simulink model "EE401_Lab_Simulation_DQ Frame"  (R2019a)
settings: Solver=VariableStepAuto  StartTime=0.0  StopTime=2  MaxStep=0.0001  RelTol=1e-3
model workspace (MAT data in the model file):
  J = 0.02
  Lm = 0.2037
  Lr = 0.2097
  Ls = 0.2097
  P = 4
  Rr = 1.083
  Rs = 1.115
  TL = 20
  We = 376.99
libraries: powerlib x1
settings Model: OrderedModelArguments=off  Creator=omkar  LastModifiedBy=omkar

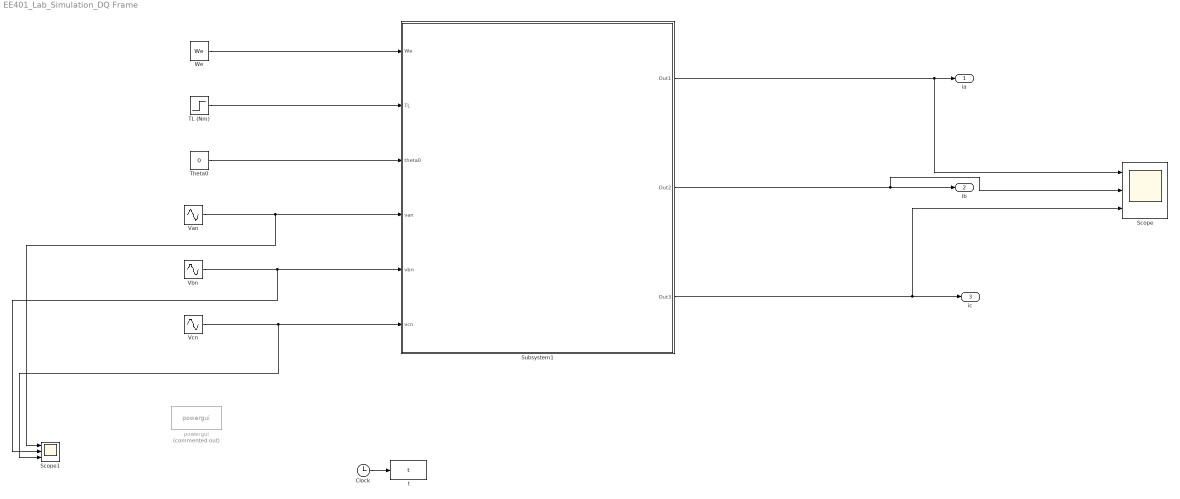
== system EE401_Lab_Simulation_DQ Frame ==
  "Clock " : Clock
  Scope : Scope  NumInputPorts=3
  Scope1 : Scope  NumInputPorts=3
  Subsystem1 : Subsystem
  TL (Nm) : Step  Time=0.2  After=TL  SampleTime=0
  Theta0 : Constant  Value=0
  Van : Sin  Amplitude=240  Frequency=2*pi*60  SampleTime=0
  Vbn : Sin  Amplitude=240  Frequency=2*pi*60  Phase=-2*pi/3  SampleTime=0
  Vcn : Sin  Amplitude=240  Frequency=2*pi*60  Phase=-4*pi/3  SampleTime=0
  We : Constant  Value=We
  powergui : powerlib/powergui  Priority=1  Commented=on  SimulationMode=Continuous  SampleTime=50e-6  frequency=60  Iterations=50  frequencyindice=60  Pbase=100e6  ErrMax=1e-4  UnitsV=kV  UnitsW=MW  buscounter=0  FunctionMessages=off  echomessages=off  EnableUseOfTLC=off  CurrentSourceSwitches=off  DisableSnubberDevices=off  DisableRonSwitches=off  DisableVfSwitches=off  DisplayEquations=off  AutomaticDiscreteSolvers=off  SolverType=Tustin/Backward Euler (TBE)  Interpol=off  ExternalGateDelay=off  methode=off  Ts=100  x0status=blocks  SPID=on  SwTol=0  HookPort=off  NonlinearTolerance=0  nMaxIteration=15  ContinueOnMaxIteration=off  RestoreLinks=warning  ResistiveCurrentMeasurement=off  Frange=[0:2:500]  Ylog=off  Xlog=on  ShowGrid=off  save=off  variable=ZData  structure=0  ZoomFFT=off  StartTime=0.0  cycles=1  DisplayStyle=1  fundamental=60  FreqAxis=off  MaxFrequency=1000  frequencyindicesteady=1  RmsSteady=1  display=off
      settings: SourceProductName=Simscape Electrical
  t : ToWorkspace  VariableName=t  SaveFormat=Timeseries  SampleTime=-1
  ia : Outport  VectorParamsAs1DForOutWhenUnconnected=on
  ib : Outport  Port=2  VectorParamsAs1DForOutWhenUnconnected=on
  ic : Outport  Port=3  VectorParamsAs1DForOutWhenUnconnected=on
  wires:
  We/1 -> Subsystem1/1(We)
  Theta0/1 -> Subsystem1/3(theta0)
  Subsystem1/1(Out1) -> Scope/1, ia/1
  Subsystem1/2(Out2) -> Scope/2, ib/1
  Subsystem1/3(Out3) -> Scope/3, ic/1
  Van/1 -> Scope1/1, Subsystem1/4(van)
  Vbn/1 -> Scope1/2, Subsystem1/5(vbn)
  Vcn/1 -> Scope1/3, Subsystem1/6(vcn)
  TL (Nm)/1 -> Subsystem1/2(TL)
  "Clock "/1 -> t/1

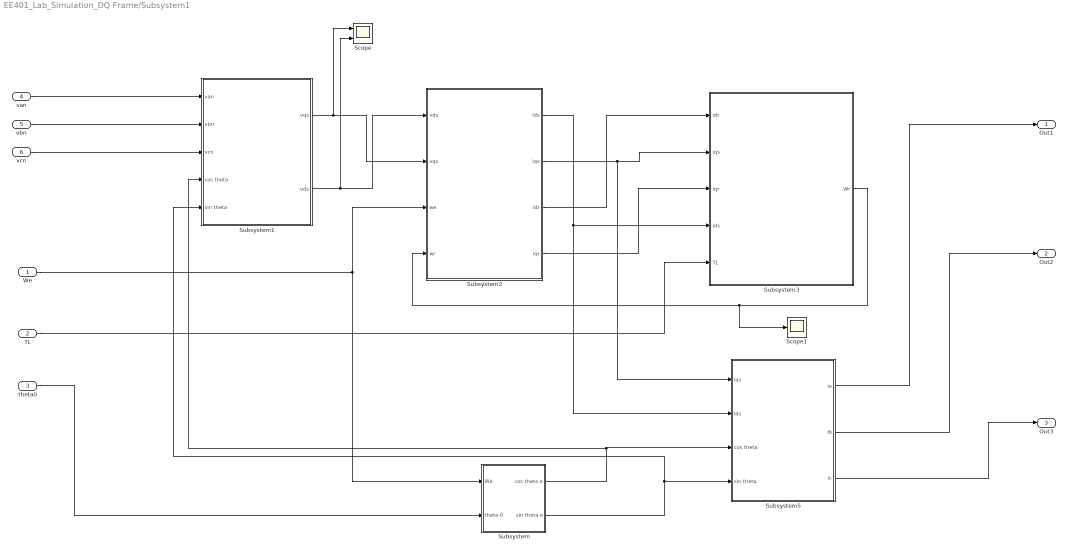
== system EE401_Lab_Simulation_DQ Frame/Subsystem1 ==
  We : Inport
  TL : Inport  Port=2
  theta0 : Inport  Port=3
  van : Inport  Port=4
  vbn : Inport  Port=5
  vcn : Inport  Port=6
  Scope : Scope  NumInputPorts=2
  Scope1 : Scope
  Subsystem : Subsystem
  Subsystem1 : Subsystem
  Subsystem2 : Subsystem
  Subsystem3 : Subsystem
  Subsystem5 : Subsystem
  Out1 : Outport
  Out2 : Outport  Port=2
  Out3 : Outport  Port=3
  wires:
  Subsystem5/3(ic) -> Out3/1
  We/1 -> Subsystem2/3(we), Subsystem/1(We)
  Subsystem2/4(iqr) -> Subsystem3/3(iqr)
  Subsystem2/3(idr) -> Subsystem3/1(idr)
  Subsystem2/1(ids) -> Subsystem5/2(ids), Subsystem3/4(ids)
  Subsystem2/2(iqs) -> Subsystem5/1(iqs), Subsystem3/2(iqs)
  Subsystem3/1(Wr) -> Scope1/1, Subsystem2/4(wr)
  Subsystem5/1(ia) -> Out1/1
  Subsystem5/2(ib) -> Out2/1
  theta0/1 -> Subsystem/2(theta 0)
  TL/1 -> Subsystem3/5(TL)
  Subsystem1/2(vds) -> Scope/2, Subsystem2/1(vds)
  Subsystem1/1(vqs) -> Scope/1, Subsystem2/2(vqs)
  van/1 -> Subsystem1/1(van)
  vbn/1 -> Subsystem1/2(vbn)
  vcn/1 -> Subsystem1/3(vcn)
  Subsystem/1(cos theta e) -> Subsystem1/4(cos theta), Subsystem5/3(cos theta)
  Subsystem/2(sin theta e) -> Subsystem5/4(sin theta), Subsystem1/5(sin theta)

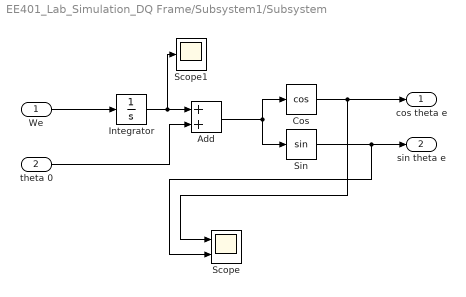
== system EE401_Lab_Simulation_DQ Frame/Subsystem1/Subsystem ==
  We : Inport
  theta 0 : Inport  Port=2
  Add : Sum
  Cos : Trigonometry  Operator=cos
  Integrator : Integrator
  Scope : Scope  NumInputPorts=2
  Scope1 : Scope
  Sin : Trigonometry
  cos theta e : Outport
  sin theta e : Outport  Port=2
  wires:
  Integrator/1 -> Scope1/1, Add/1
  Add/1 -> Cos/1, Sin/1
  theta 0/1 -> Add/2
  Sin/1 -> Scope/2, sin theta e/1
  We/1 -> Integrator/1
  Cos/1 -> Scope/1, cos theta e/1

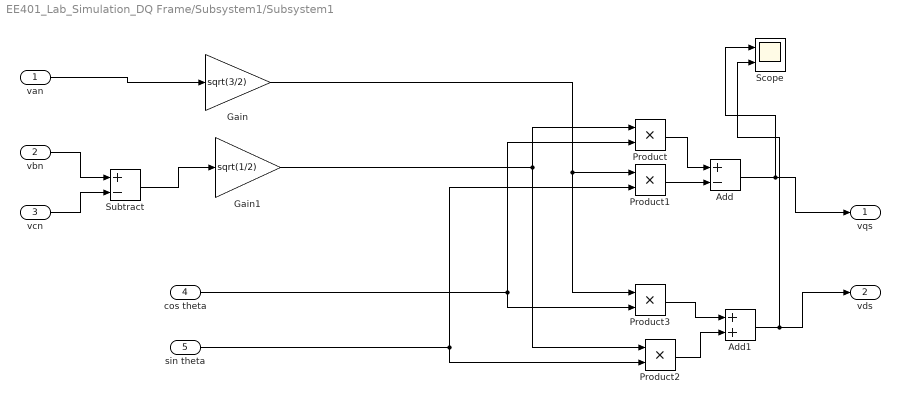
== system EE401_Lab_Simulation_DQ Frame/Subsystem1/Subsystem1 ==
  van : Inport
  vbn : Inport  Port=2
  vcn : Inport  Port=3
  cos theta : Inport  Port=4
  sin theta : Inport  Port=5
  Add : Sum  Inputs=+-
  Add1 : Sum
  Gain : Gain  Gain=sqrt(3/2)
  Gain1 : Gain  Gain=sqrt(1/2)
  Product{,1..3} (4 alike) : Product
  Scope : Scope  NumInputPorts=2
  Subtract : Sum  Inputs=+-
  vqs : Outport
  vds : Outport  Port=2
  wires:
  van/1 -> Gain/1
  sin theta/1 -> Product2/2, Product1/2
  Product1/1 -> Add/2
  cos theta/1 -> Product/2, Product3/2
  Gain/1 -> Product1/1, Product3/1
  Product2/1 -> Add1/2
  Product3/1 -> Add1/1
  Product/1 -> Add/1
  Gain1/1 -> Product/1, Product2/1
  vbn/1 -> Subtract/1
  vcn/1 -> Subtract/2
  Add/1 -> Scope/1, vqs/1
  Add1/1 -> Scope/2, vds/1
  Subtract/1 -> Gain1/1

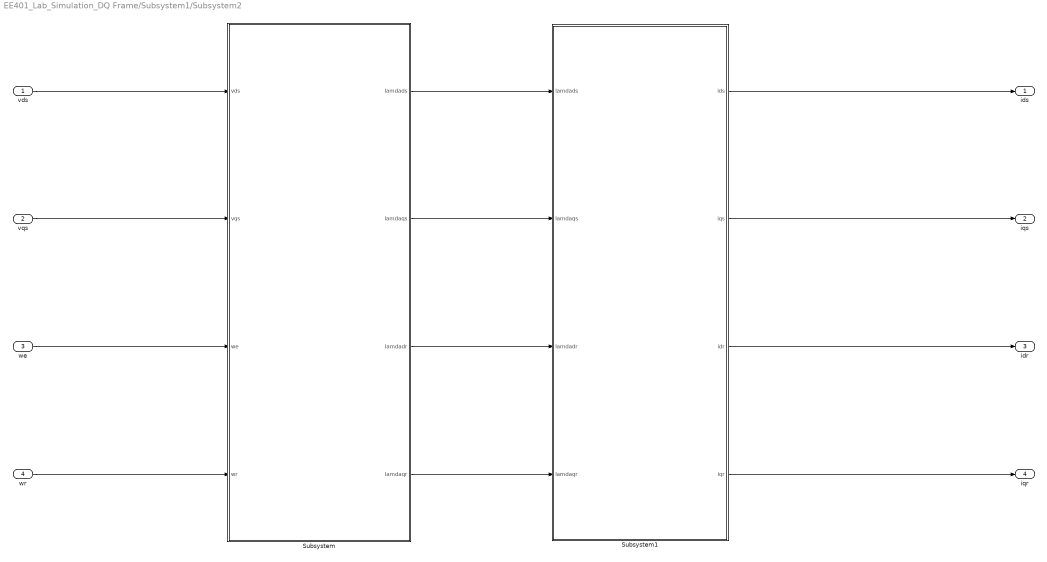
== system EE401_Lab_Simulation_DQ Frame/Subsystem1/Subsystem2 ==
  vds : Inport
  vqs : Inport  Port=2
  we : Inport  Port=3
  wr : Inport  Port=4
  Subsystem : Subsystem
  Subsystem1 : Subsystem
  ids : Outport
  iqs : Outport  Port=2
  idr : Outport  Port=3
  iqr : Outport  Port=4
  wires:
  wr/1 -> Subsystem/4(wr)
  Subsystem1/3(idr) -> idr/1
  Subsystem/4(lamdaqr) -> Subsystem1/4(lamdaqr)
  Subsystem/3(lamdadr) -> Subsystem1/3(lamdadr)
  Subsystem/1(lamdads) -> Subsystem1/1(lamdads)
  we/1 -> Subsystem/3(we)
  Subsystem/2(lamdaqs) -> Subsystem1/2(lamdaqs)
  Subsystem1/4(iqr) -> iqr/1
  Subsystem1/1(ids) -> ids/1
  Subsystem1/2(iqs) -> iqs/1
  vds/1 -> Subsystem/1(vds)
  vqs/1 -> Subsystem/2(vqs)

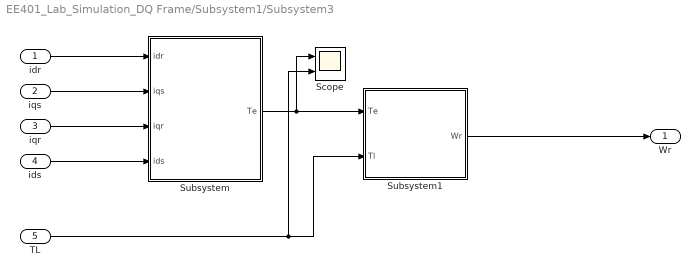
== system EE401_Lab_Simulation_DQ Frame/Subsystem1/Subsystem3 ==
  idr : Inport
  iqs : Inport  Port=2
  iqr : Inport  Port=3
  ids : Inport  Port=4
  TL : Inport  Port=5
  Scope : Scope  NumInputPorts=2
  Subsystem : Subsystem
  Subsystem1 : Subsystem
  Wr : Outport
  wires:
  ids/1 -> Subsystem/4(ids)
  iqr/1 -> Subsystem/3(iqr)
  Subsystem/1(Te) -> Scope/1, Subsystem1/1(Te)
  idr/1 -> Subsystem/1(idr)
  Subsystem1/1(Wr) -> Wr/1
  TL/1 -> Scope/2, Subsystem1/2(Tl)
  iqs/1 -> Subsystem/2(iqs)

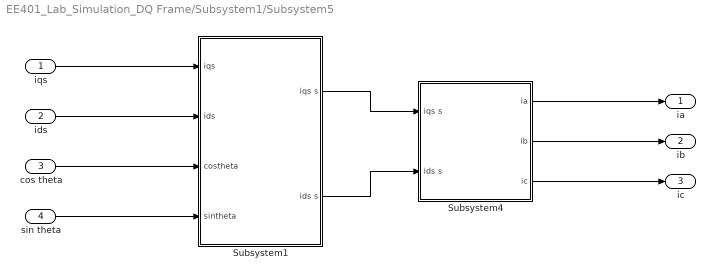
== system EE401_Lab_Simulation_DQ Frame/Subsystem1/Subsystem5 ==
  iqs : Inport
  ids : Inport  Port=2
  cos theta : Inport  Port=3
  sin theta : Inport  Port=4
  Subsystem1 : Subsystem
  Subsystem4 : Subsystem
  ia : Outport
  ib : Outport  Port=2
  ic : Outport  Port=3
  wires:
  sin theta/1 -> Subsystem1/4(sintheta)
  Subsystem1/1(iqs s) -> Subsystem4/1(iqs s)
  Subsystem4/1(ia) -> ia/1
  Subsystem4/3(ic) -> ic/1
  ids/1 -> Subsystem1/2(ids)
  cos theta/1 -> Subsystem1/3(costheta)
  Subsystem4/2(ib) -> ib/1
  Subsystem1/2(ids s) -> Subsystem4/2(ids s)
  iqs/1 -> Subsystem1/1(iqs)

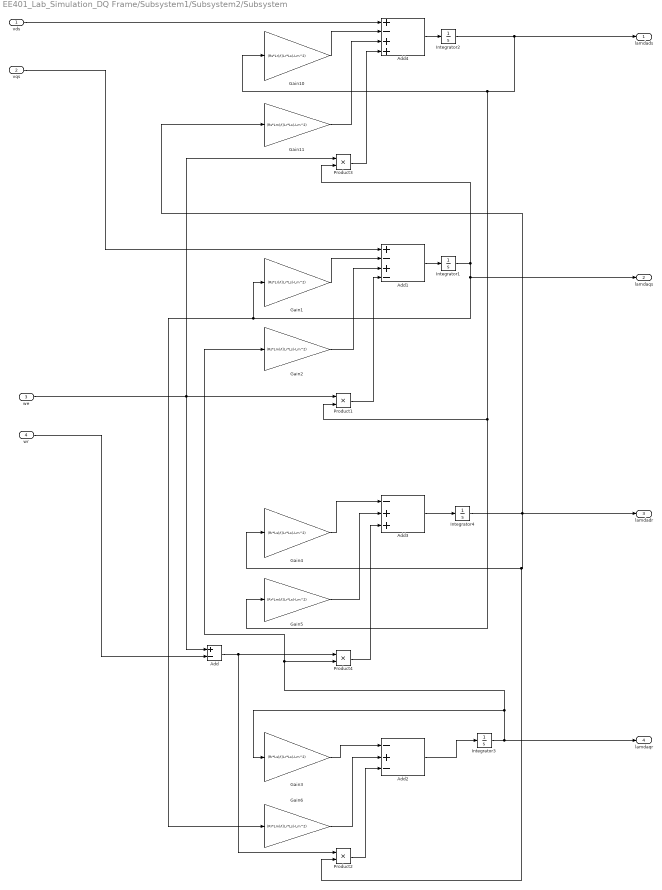
== system EE401_Lab_Simulation_DQ Frame/Subsystem1/Subsystem2/Subsystem ==
  vds : Inport
  vqs : Inport  Port=2
  we : Inport  Port=3
  wr : Inport  Port=4
  Add : Sum  Inputs=+-
  Add1 : Sum  Inputs=+-+-
  Add2 : Sum  Inputs=-+-
  Add3 : Sum  Inputs=-++
  Add4 : Sum  Inputs=+-++
  Gain1 : Gain  Gain=(Rs*Lr)/((Lr*Ls)-Lm^2)
  Gain10 : Gain  Gain=(Rs*Lr)/((Lr*Ls)-Lm^2)
  Gain11 : Gain  Gain=(Rs*Lm)/((Lr*Ls)-Lm^2)
  Gain2 : Gain  Gain=(Rs*Lm)/((Lr*Ls)-Lm^2)
  Gain3 : Gain  Gain=(Rr*Ls)/((Lr*Ls)-Lm^2)
  Gain4 : Gain  Gain=(Rr*Ls)/((Lr*Ls)-Lm^2)
  Gain5 : Gain  Gain=(Rr*Lm)/((Lr*Ls)-Lm^2)
  Gain6 : Gain  Gain=(Rr*Lm)/((Lr*Ls)-Lm^2)
  Integrator{1..4} (4 alike) : Integrator
  Product{1..4} (4 alike) : Product
  lamdads : Outport
  lamdaqs : Outport  Port=2
  lamdadr : Outport  Port=3
  lamdaqr : Outport  Port=4
  wires:
  Gain4/1 -> Add3/1
  Gain3/1 -> Add2/1
  Gain2/1 -> Add1/3
  Product2/1 -> Add2/3
  vqs/1 -> Add1/1
  Integrator1/1 -> lamdaqs/1, Gain6/1, Gain1/1, Product3/2
  Integrator2/1 -> lamdads/1, Gain10/1, Gain5/1, Product1/2
  we/1 -> Product3/1, Add/1, Product1/1
  Gain5/1 -> Add3/2
  Gain11/1 -> Add4/3
  Integrator4/1 -> Gain11/1, lamdadr/1, Product2/2, Gain4/1
  Product4/1 -> Add3/3
  Add2/1 -> Integrator3/1
  Gain6/1 -> Add2/2
  Add4/1 -> Integrator2/1
  Integrator3/1 -> lamdaqr/1, Gain2/1, Product4/2, Gain3/1
  Add3/1 -> Integrator4/1
  wr/1 -> Add/2
  Gain1/1 -> Add1/2
  Add1/1 -> Integrator1/1
  Product1/1 -> Add1/4
  Product3/1 -> Add4/4
  Gain10/1 -> Add4/2
  Add/1 -> Product4/1, Product2/1
  vds/1 -> Add4/1

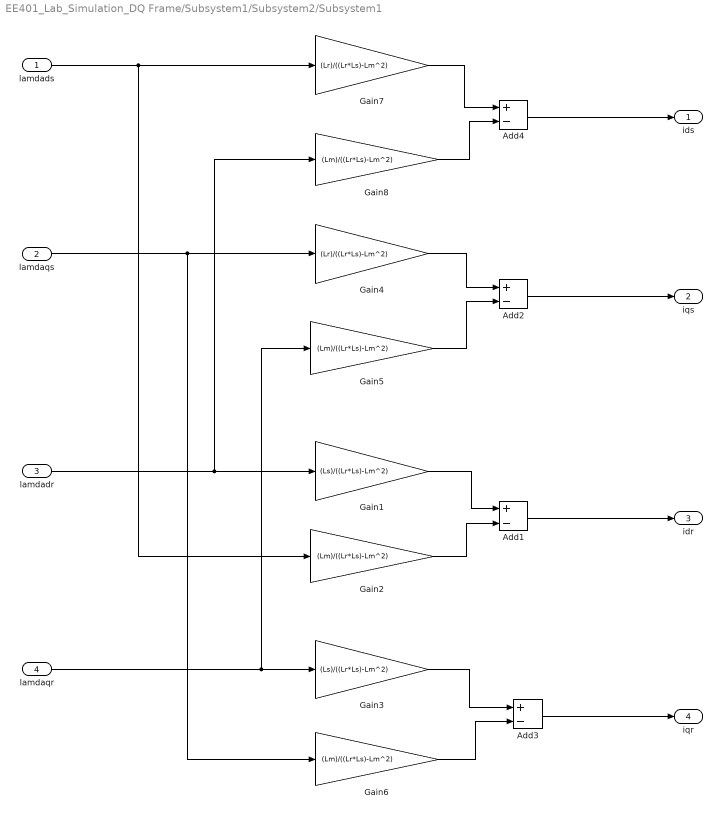
== system EE401_Lab_Simulation_DQ Frame/Subsystem1/Subsystem2/Subsystem1 ==
  lamdads : Inport
  lamdaqs : Inport  Port=2
  lamdadr : Inport  Port=3
  lamdaqr : Inport  Port=4
  Add{1..4} (4 alike) : Sum  Inputs=+-
  Gain1 : Gain  Gain=(Ls)/((Lr*Ls)-Lm^2)
  Gain{2,5..6,8} (4 alike) : Gain  Gain=(Lm)/((Lr*Ls)-Lm^2)
  Gain3 : Gain  Gain=(Ls)/((Lr*Ls)-Lm^2)
  Gain4 : Gain  Gain=(Lr)/((Lr*Ls)-Lm^2)
  Gain7 : Gain  Gain=(Lr)/((Lr*Ls)-Lm^2)
  ids : Outport
  iqs : Outport  Port=2
  idr : Outport  Port=3
  iqr : Outport  Port=4
  wires:
  Gain1/1 -> Add1/1
  Gain2/1 -> Add1/2
  Gain4/1 -> Add2/1
  Gain8/1 -> Add4/2
  Gain7/1 -> Add4/1
  Gain5/1 -> Add2/2
  lamdadr/1 -> Gain1/1, Gain8/1
  lamdaqs/1 -> Gain6/1, Gain4/1
  lamdaqr/1 -> Gain5/1, Gain3/1
  Add4/1 -> ids/1
  lamdads/1 -> Gain2/1, Gain7/1
  Gain6/1 -> Add3/2
  Gain3/1 -> Add3/1
  Add2/1 -> iqs/1
  Add1/1 -> idr/1
  Add3/1 -> iqr/1

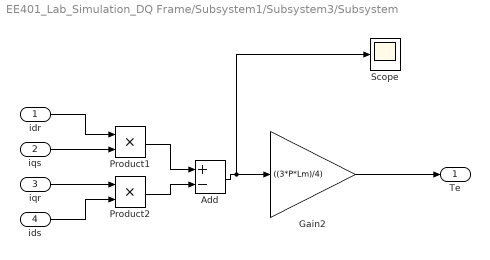
== system EE401_Lab_Simulation_DQ Frame/Subsystem1/Subsystem3/Subsystem ==
  idr : Inport
  iqs : Inport  Port=2
  iqr : Inport  Port=3
  ids : Inport  Port=4
  Add : Sum  Inputs=+-
  Gain2 : Gain  Gain=((3*P*Lm)/4)
  Product1 : Product
  Product2 : Product
  Scope : Scope
  Te : Outport
  wires:
  Product2/1 -> Add/2
  Product1/1 -> Add/1
  iqs/1 -> Product1/2
  iqr/1 -> Product2/1
  Gain2/1 -> Te/1
  Add/1 -> Scope/1, Gain2/1
  ids/1 -> Product2/2
  idr/1 -> Product1/1

== system EE401_Lab_Simulation_DQ Frame/Subsystem1/Subsystem3/Subsystem1 ==
  Te : Inport
  Tl : Inport  Port=2
  Add3 : Sum  Inputs=+-
  Gain6 : Gain  Gain=(P)/(2*J)
  Integrator1 : Integrator
  Scope1 : Scope  NumInputPorts=2
  Wr : Outport
  wires:
  Tl/1 -> Scope1/2, Add3/2
  Add3/1 -> Gain6/1
  Gain6/1 -> Integrator1/1
  Integrator1/1 -> Wr/1
  Te/1 -> Scope1/1, Add3/1

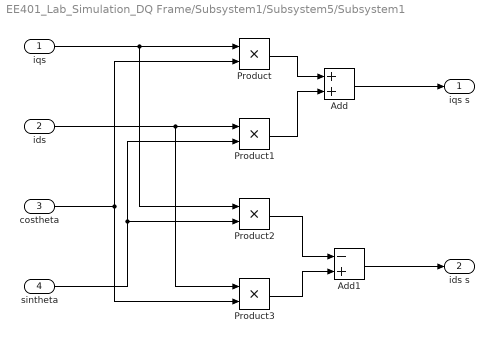
== system EE401_Lab_Simulation_DQ Frame/Subsystem1/Subsystem5/Subsystem1 ==
  iqs : Inport
  ids : Inport  Port=2
  costheta : Inport  Port=3
  sintheta : Inport  Port=4
  Add : Sum
  Add1 : Sum  Inputs=-+
  Product{,1..3} (4 alike) : Product
  iqs s : Outport
  ids s : Outport  Port=2
  wires:
  Product3/1 -> Add1/2
  costheta/1 -> Product/2, Product3/2
  sintheta/1 -> Product2/2, Product1/2
  Add/1 -> iqs s/1
  Product2/1 -> Add1/1
  iqs/1 -> Product2/1, Product/1
  Product1/1 -> Add/2
  Product/1 -> Add/1
  ids/1 -> Product3/1, Product1/1
  Add1/1 -> ids s/1

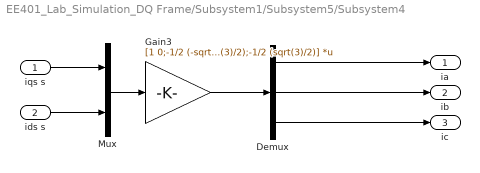
== system EE401_Lab_Simulation_DQ Frame/Subsystem1/Subsystem5/Subsystem4 ==
  iqs s : Inport
  ids s : Inport  Port=2
  Demux : Demux  Outputs=3
  Gain3 : Gain  Gain=[1 0;-1/2 (-sqrt(3)/2);-1/2 (sqrt(3)/2)]  Multiplication=Matrix(K*u)
  Mux : Mux  Inputs=2
  ia : Outport
  ib : Outport  Port=2
  ic : Outport  Port=3
  wires:
  Demux/2 -> ib/1
  Gain3/1 -> Demux/1
  Mux/1 -> Gain3/1
  Demux/1 -> ia/1
  Demux/3 -> ic/1
  iqs s/1 -> Mux/1
  ids s/1 -> Mux/2
